simulink model "multirotorPathDynamics"  (R2021b)
settings: Solver=VariableStepAuto  StartTime=0.0  StopTime=210  RelTol=1e-3
InitFcn:
  | FidelityStage = 2;
model workspace (MAT data in the model file):
  airspeedVal = 52.6655095712
  lastWaypointInstance = [-815.416609718; 1327.32979057; -188.3664]
  waypointData = [-1257.59078698 -1257.11235464 -1256.63393535 -1256.15552911 -1255.67713593 -1255.19875581 -1254.72038874 -1254.24203473 -1253.76369377 -1253.28536587 -1252.8070545 -1252.32876157 ... (1797 elements, 599x3)]
undefined symbols (not defined in the file): DroneMass, Dz, Earth, Gravity, Iz, Nz, Pz, startFlightTime, UAVSampleTime, WGS84
libraries: slpidlib x6, uavalgslib x2, aerolibconvert2 x1, aerolibtransform2 x1
(part 1 of 2)
settings Model: DataDictionary=multirotorPathDataDict.sldd  PauseTimes=120  Creator=IRC  LastModifiedBy=IRC
settings DataIOCC: SaveState=on  ReturnWorkspaceOutputs=off
settings DebuggingCC: UnderSpecifiedDataTypeMsg=warning  UnderSpecifiedDimensionMsg=warning

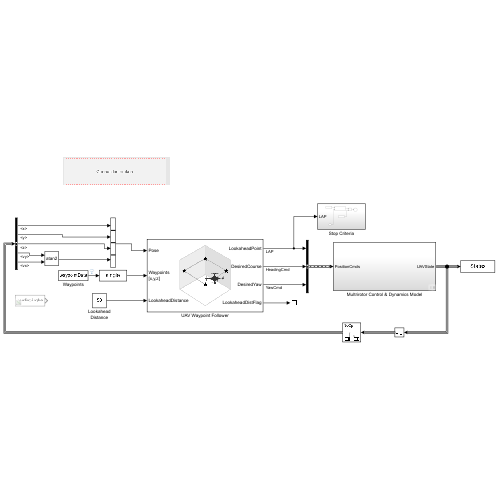
[thumbnail: Simulink's stored preview of the top-level diagram]
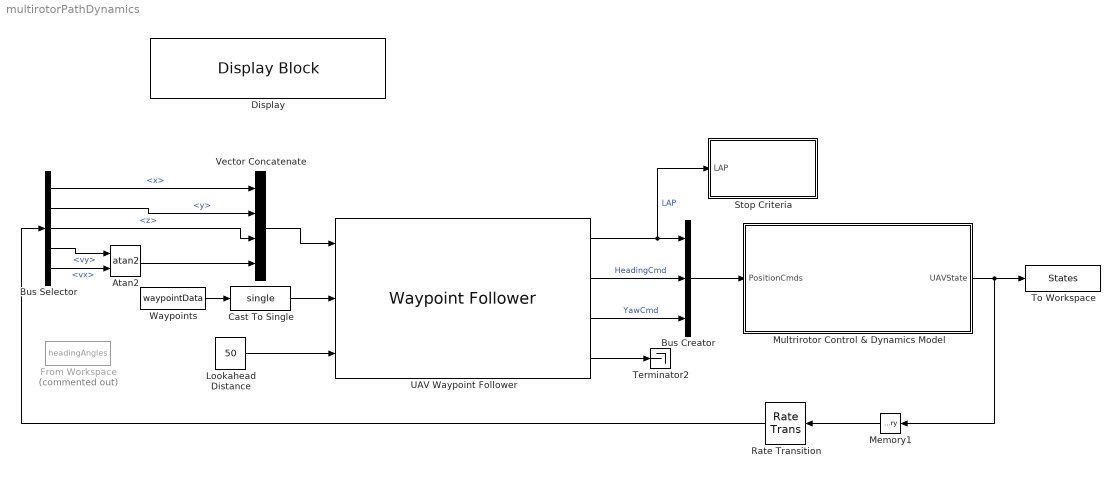
== system multirotorPathDynamics ==
  Atan2 : Trigonometry  Operator=atan2
  Bus Creator : BusCreator  Inputs=3  OutDataTypeStr=Bus: innerLoopCmdsBus  NonVirtualBus=on
  Bus Selector : BusSelector  OutputSignals=pos_vel.x,pos_vel.y,pos_vel.z,pos_vel.vy,pos_vel.vx
  Cast To Single : DataTypeConversion  OutDataTypeStr=single
  Display : DisplayBlock  Format=short  Transparency=1
  From Workspace : FromWorkspace  Commented=on  VariableName=headingAngles  SampleTime=-1
  Lookahead Distance : Constant  Value=50  OutDataTypeStr=single
  Memory1 : Memory  InheritSampleTime=on
  Multrirotor Control & Dynamics Model : Subsystem  VariantControl=plantModelFi ==0
  Rate Transition : RateTransition
  Stop Criteria : Subsystem
  Terminator2 : Terminator
  To Workspace : ToWorkspace  VariableName=States  SaveFormat=Timeseries  SampleTime=-1
  UAV Waypoint Follower : uavalgslib/Waypoint Follower  UAVType=multirotor  StartFrom=first  TransitionRadiusSource=internal  TransitionRadius=10  MinLookaheadDistance=0.1  YawInput=off  ShowCrossTrackErrorOutput=off  ShowStatusOutput=off  SimulateUsing=Code generation
      settings: SourceProductBaseCode=UV
  Vector Concatenate : Concatenate  NumInputs=4
  Waypoints : Constant  Value=waypointData  VectorParams1D=off
  wires:
  UAV Waypoint Follower/1 -> Stop Criteria/1(LAP), Bus Creator/1  "LAP"
  UAV Waypoint Follower/2 -> Bus Creator/2  "HeadingCmd"
  UAV Waypoint Follower/3 -> Bus Creator/3  "YawCmd"
  Lookahead Distance/1 -> UAV Waypoint Follower/3
  Bus Selector/1 -> Vector Concatenate/1  "<x>"
  Bus Selector/2 -> Vector Concatenate/2  "<y>"
  UAV Waypoint Follower/4 -> Terminator2/1
  Waypoints/1 -> Cast To Single/1
  Cast To Single/1 -> UAV Waypoint Follower/2
  Bus Selector/3 -> Vector Concatenate/3  "<z>"
  Vector Concatenate/1 -> UAV Waypoint Follower/1
  Memory1/1 -> Rate Transition/1
  Rate Transition/1 -> Bus Selector/1
  Bus Selector/4 -> Atan2/1  "<vy>"
  Bus Selector/5 -> Atan2/2  "<vx>"
  Atan2/1 -> Vector Concatenate/4
  Bus Creator/1 -> Multrirotor Control & Dynamics Model/1(PositionCmds)
  Multrirotor Control & Dynamics Model/1(UAVState) -> To Workspace/1, Memory1/1

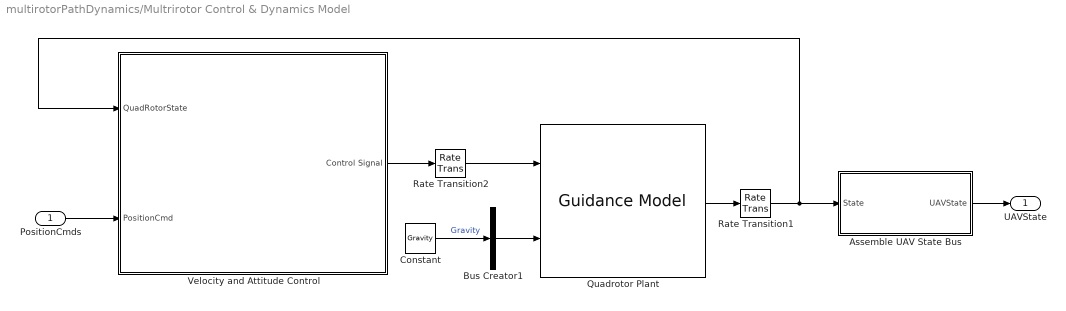
== system multirotorPathDynamics/Multrirotor Control & Dynamics Model ==
  PositionCmds : Inport
  Assemble UAV State Bus : Subsystem
  Bus Creator1 : BusCreator  Inputs=1  OutDataTypeStr=Bus: uavGuidanceEnvironmentBus  NonVirtualBus=on
  Constant : Constant  Value=Gravity  OutDataTypeStr=single
      settings: AttributesFormatString=%<Value>
  Quadrotor Plant : uavalgslib/Guidance Model  ModelType=MultirotorGuidance  SpecifiedDataType=single  SimulateUsing=Code generation  InitialWorldPositionMultirotor=initialConditions.posNED'  InitialWorldVelocityMultirotor=initialConditions.vb'  InitialEulerZYXMultirotor=[0; 0; 0]  InitialBodyAngularRateRPYMultirotor=[0; 0; 0]  InitialThrustMultirotor=0  InitialNorthFixedWing=0  InitialEastFixedWing=0  InitialHeightFixedWing=0  InitialAirSpeedFixedWing=0  InitialHeadingAngleFixedWing=0  InitialFlightPathAngleFixedWing=0  InitialRollAngleFixedWing=0  InitialRollAngleRateFixedWing=0  PDRollMultirotor=[3402.97,116.67]  PDPitchMultirotor=[3402.97, 116.67]  PYawRateMultirotor=1950  PThrustMultirotor=39  MassMultirotor=0.1  PHeightFixedWing=3.9  PHeadingAngleFixedWing=3.9  PFlightPathAngleFixedWing=39  PDRollFixedWing=[3402.97, 116.67]  PAirSpeedFixedWing=1  FlightPathAngleLimitsFixedWing=[-pi/2, pi/2]  StateBusName='uavGuidanceStateBus'  ControlBusName='uavGuidanceControlBus'  EnvironmentBusName='uavGuidanceEnvironmentBus'  DataType=single
      settings: SourceProductName=UAV Toolbox
  Rate Transition1 : RateTransition  OutPortSampleTime=UAVSampleTime
  Rate Transition2 : RateTransition  OutPortSampleTime=UAVSampleTime
  Velocity and Attitude Control : Subsystem
  UAVState : Outport  OutDataTypeStr=Bus: uavStateBus
  wires:
  Constant/1 -> Bus Creator1/1  "Gravity"
  Bus Creator1/1 -> Quadrotor Plant/2
  Velocity and Attitude Control/1(Control Signal) -> Rate Transition2/1
  Quadrotor Plant/1 -> Rate Transition1/1
  Rate Transition2/1 -> Quadrotor Plant/1
  PositionCmds/1 -> Velocity and Attitude Control/2(PositionCmd)
  Rate Transition1/1 -> Velocity and Attitude Control/1(QuadRotorState), Assemble UAV State Bus/1(State)
  Assemble UAV State Bus/1(UAVState) -> UAVState/1

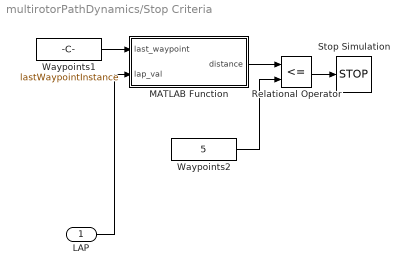
== system multirotorPathDynamics/Stop Criteria ==
  LAP : Inport
  MATLAB Function : MATLAB Function  TreatAsAtomicUnit=on
  Relational Operator : RelationalOperator  Operator=<=  OutDataTypeStr=boolean  RndMeth=Simplest
  Stop Simulation : Stop
  Waypoints1 : Constant  Value=lastWaypointInstance  VectorParams1D=off
  Waypoints2 : Constant  Value=5  VectorParams1D=off
  wires:
  MATLAB Function/1(distance) -> Relational Operator/1
  Waypoints2/1 -> Relational Operator/2
  Waypoints1/1 -> MATLAB Function/1(last_waypoint)
  Relational Operator/1 -> Stop Simulation/1
  LAP/1 -> MATLAB Function/2(lap_val)

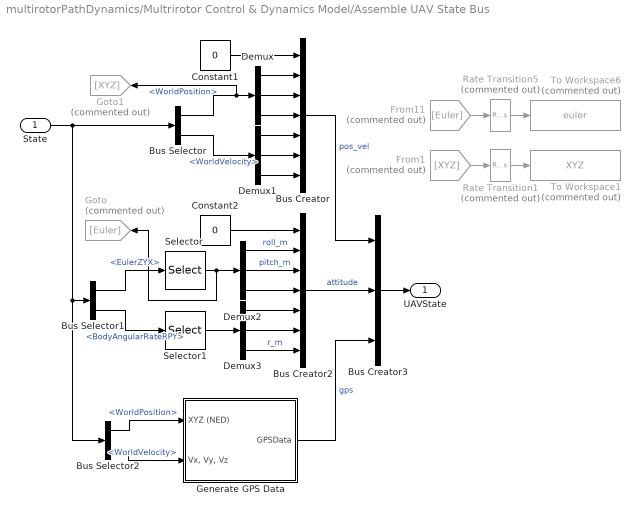
== system multirotorPathDynamics/Multrirotor Control & Dynamics Model/Assemble UAV State Bus ==
  State : Inport
  Bus Creator : BusCreator  Inputs=7  OutDataTypeStr=Bus: local_position_ned
      settings: InheritFromInputs=off
  Bus Creator2 : BusCreator  Inputs=7  OutDataTypeStr=Bus: attitudeBus
      settings: InheritFromInputs=off
  Bus Creator3 : BusCreator  Inputs=3  OutDataTypeStr=Bus: uavStateBus
      settings: InheritFromInputs=off
  Bus Selector : BusSelector  OutputSignals=WorldPosition,WorldVelocity
  Bus Selector1 : BusSelector  OutputSignals=EulerZYX,BodyAngularRateRPY
  Bus Selector2 : BusSelector  OutputSignals=WorldPosition,WorldVelocity
  Constant1 : Constant  Value=0  OutDataTypeStr=uint32
  Constant2 : Constant  Value=0  OutDataTypeStr=uint32
  Demux{,1..3} (4 alike) : Demux  Outputs=3
  From1 : From  Commented=on  GotoTag=XYZ
  From11 : From  Commented=on  GotoTag=Euler
  Generate GPS Data : Subsystem
  Goto : Goto  Commented=on  GotoTag=Euler
  Goto1 : Goto  Commented=on  GotoTag=XYZ
  Rate Transition1 : RateTransition  Commented=on  OutPortSampleTime=UAVSampleTime
  Rate Transition5 : RateTransition  Commented=on  OutPortSampleTime=UAVSampleTime
  Selector : Selector  InputPortWidth=3  IndexOptions=Index vector (dialog)  Indices=[3 2 1]  OutputSizes=1
  Selector1 : Selector  InputPortWidth=3  IndexOptions=Index vector (dialog)  Indices=[3 2 1]  OutputSizes=1
  To Workspace1 : ToWorkspace  Commented=on  VariableName=XYZ  SaveFormat=Timeseries  SampleTime=-1
  To Workspace6 : ToWorkspace  Commented=on  VariableName=euler  SaveFormat=Timeseries  SampleTime=-1
  UAVState : Outport  OutDataTypeStr=Bus: uavStateBus
  wires:
  Bus Creator2/1 -> Bus Creator3/2  "attitude"
  Bus Creator3/1 -> UAVState/1
  Demux3/1 -> Bus Creator2/5
  Demux1/2 -> Bus Creator/6
  Bus Creator/1 -> Bus Creator3/1  "pos_vel"
  Demux1/3 -> Bus Creator/7
  Bus Selector2/2 -> Generate GPS Data/2("Vx, Vy, Vz")  "<WorldVelocity>"
  Demux/1 -> Bus Creator/2
  State/1 -> Bus Selector/1, Bus Selector2/1, Bus Selector1/1
  Constant2/1 -> Bus Creator2/1
  Bus Selector/1 -> Goto1/1, Demux/1  "<WorldPosition>"
  Selector1/1 -> Demux3/1
  Demux1/1 -> Bus Creator/5
  Bus Selector1/1 -> Selector/1  "<EulerZYX>"
  Demux/2 -> Bus Creator/3
  Demux2/1 -> Bus Creator2/2  "roll_m"
  Demux2/3 -> Bus Creator2/4
  Demux3/2 -> Bus Creator2/6
  Demux2/2 -> Bus Creator2/3  "pitch_m"
  Bus Selector1/2 -> Selector1/1  "<BodyAngularRateRPY>"
  Demux3/3 -> Bus Creator2/7  "r_m"
  Demux/3 -> Bus Creator/4
  Bus Selector/2 -> Demux1/1  "<WorldVelocity>"
  Constant1/1 -> Bus Creator/1
  Bus Selector2/1 -> Generate GPS Data/1(XYZ (NED))  "<WorldPosition>"
  Generate GPS Data/1(GPSData) -> Bus Creator3/3  "gps"
  Rate Transition5/1 -> To Workspace6/1
  From11/1 -> Rate Transition5/1
  Selector/1 -> Goto/1, Demux2/1
  From1/1 -> Rate Transition1/1
  Rate Transition1/1 -> To Workspace1/1

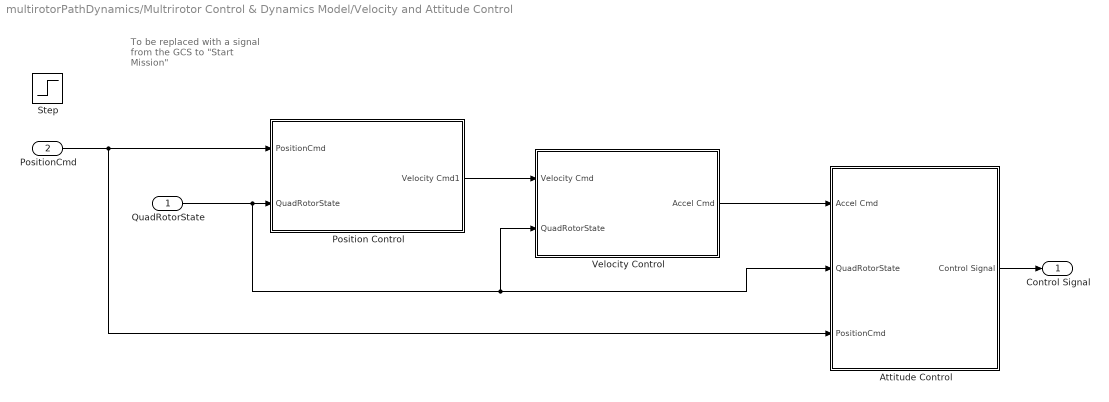
== system multirotorPathDynamics/Multrirotor Control & Dynamics Model/Velocity and Attitude Control ==
  note: To be replaced with a signal from the GCS to "Start Mission"
  QuadRotorState : Inport
  PositionCmd : Inport  Port=2
  Attitude Control : Subsystem
  Position Control : Subsystem
  Step : Step  Time=startFlightTime  SampleTime=UAVSampleTime
  Velocity Control : Subsystem
  Control Signal : Outport
  wires:
  PositionCmd/1 -> Position Control/1(PositionCmd), Attitude Control/3(PositionCmd)
  Velocity Control/1(Accel Cmd) -> Attitude Control/1(Accel Cmd)
  Attitude Control/1(Control Signal) -> Control Signal/1
  QuadRotorState/1 -> Velocity Control/2(QuadRotorState), Attitude Control/2(QuadRotorState), Position Control/2(QuadRotorState)
  Position Control/1(Velocity Cmd1) -> Velocity Control/1(Velocity Cmd)

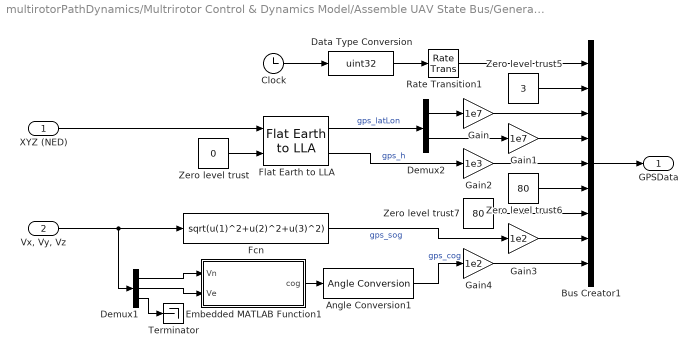
== system multirotorPathDynamics/Multrirotor Control & Dynamics Model/Assemble UAV State Bus/Generate GPS Data ==
  XYZ (NED) : Inport
  "Vx, Vy, Vz" : Inport  Port=2
  Angle Conversion1 : aerolibconvert2/Angle Conversion  IU=rad  OU=deg
  Bus Creator1 : BusCreator  Inputs=9  OutDataTypeStr=Bus: gps_raw_int  NonVirtualBus=on
      settings: InheritFromInputs=off
  Clock : Clock
      settings: AttributesFormatString=Decimation: %<Decimation>
  Data Type Conversion : DataTypeConversion  OutDataTypeStr=uint32
  Demux1 : Demux  Outputs=3
  Demux2 : Demux  Outputs=2
  Embedded MATLAB Function1 : MATLAB Function  TreatAsAtomicUnit=on
  Fcn : Fcn  Expr=sqrt(u(1)^2+u(2)^2+u(3)^2)
  Flat Earth to LLA : aerolibtransform2/Flat Earth to LLA  units=Metric (MKS)  ptype=Earth (WGS84)  F=1/298.257223563  R=6378137  refPosPort=off  LL0=uavIC_latLon  psi=0
  Gain : Gain  Gain=1e7  OutDataTypeStr=int32
  Gain1 : Gain  Gain=1e7  OutDataTypeStr=int32
  Gain2 : Gain  Gain=1e3  OutDataTypeStr=int32
  Gain3 : Gain  Gain=1e2  OutDataTypeStr=uint16
  Gain4 : Gain  Gain=1e2  OutDataTypeStr=uint16
  Rate Transition1 : RateTransition  OutPortSampleTime=UAVSampleTime
  Terminator : Terminator
  Zero level trust : Constant  Value=0
      settings: AttributesFormatString=%<Value>
  Zero level trust5 : Constant  Value=3  OutDataTypeStr=uint8
      settings: AttributesFormatString=%<Value>
  Zero level trust6 : Constant  Value=80  OutDataTypeStr=uint16
      settings: AttributesFormatString=%<Value>
  Zero level trust7 : Constant  Value=80  OutDataTypeStr=uint16
      settings: AttributesFormatString=%<Value>
  GPSData : Outport  VectorParamsAs1DForOutWhenUnconnected=off
  wires:
  Demux1/3 -> Terminator/1
  Angle Conversion1/1 -> Gain4/1  "gps_cog"
  Embedded MATLAB Function1/1(cog) -> Angle Conversion1/1
  "Vx, Vy, Vz"/1 -> Demux1/1, Fcn/1
  Demux1/2 -> Embedded MATLAB Function1/2(Ve)
  Demux1/1 -> Embedded MATLAB Function1/1(Vn)
  Fcn/1 -> Gain3/1  "gps_sog"
  Flat Earth to LLA/1 -> Demux2/1  "gps_latLon"
  Zero level trust/1 -> Flat Earth to LLA/2
  XYZ (NED)/1 -> Flat Earth to LLA/1
  Clock/1 -> Data Type Conversion/1
  Flat Earth to LLA/2 -> Gain2/1  "gps_h"
  Demux2/1 -> Gain/1
  Demux2/2 -> Gain1/1
  Zero level trust5/1 -> Bus Creator1/2
  Gain1/1 -> Bus Creator1/4
  Zero level trust6/1 -> Bus Creator1/6
  Gain3/1 -> Bus Creator1/8
  Zero level trust7/1 -> Bus Creator1/7
  Gain4/1 -> Bus Creator1/9
  Gain2/1 -> Bus Creator1/5
  Gain/1 -> Bus Creator1/3
  Data Type Conversion/1 -> Rate Transition1/1
  Bus Creator1/1 -> GPSData/1
  Rate Transition1/1 -> Bus Creator1/1

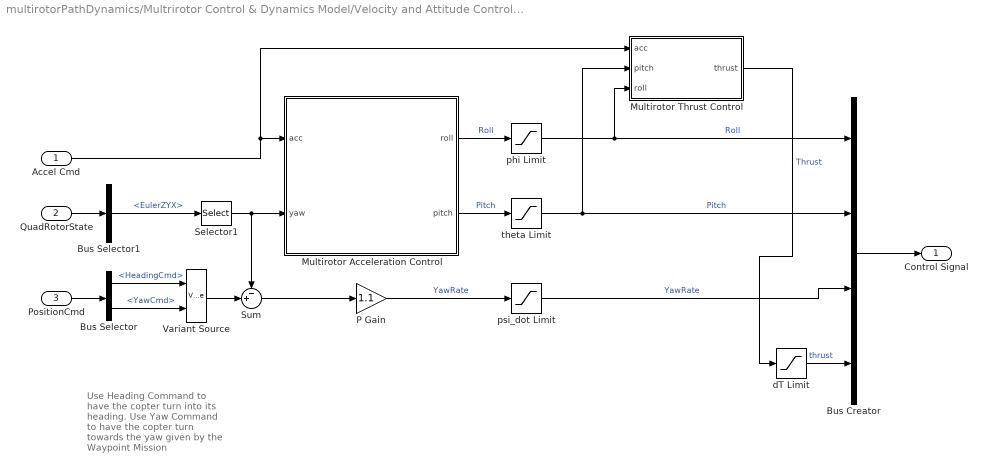
== system multirotorPathDynamics/Multrirotor Control & Dynamics Model/Velocity and Attitude Control/Attitude Control ==
  note: Use Heading Command to have
      | the copter turn into its heading.
      | Use Yaw Command to have the
      | copter turn towards the yaw given
      | by the Waypoint Mission
  Accel Cmd : Inport
  QuadRotorState : Inport  Port=2
  PositionCmd : Inport  Port=3
  Bus Creator : BusCreator  Inputs=4  OutDataTypeStr=Bus: uavGuidanceControlBus  NonVirtualBus=on
      settings: InheritFromInputs=off
  Bus Selector : BusSelector  OutputSignals=HeadingCmd,YawCmd
  Bus Selector1 : BusSelector  OutputSignals=EulerZYX
  Multirotor Acceleration Control : MATLAB Function  TreatAsAtomicUnit=on
  Multirotor Thrust Control : MATLAB Function  TreatAsAtomicUnit=on
  P Gain : Gain  Gain=1.1
  Selector1 : Selector  InputPortWidth=3  IndexOptions=Index vector (dialog)  Indices=[1]  OutputSizes=1
  Sum : Sum  Inputs=-+|
  Variant Source : VariantSource
  dT Limit : Saturate  UpperLimit=1.2  LowerLimit=0
      settings: AttributesFormatString=[%<UpperLimit> %<LowerLimit>]
  phi Limit : Saturate  UpperLimit=25*pi/180  LowerLimit=-25*pi/180
      settings: AttributesFormatString=[%<UpperLimit> %<LowerLimit>]
  psi_dot Limit : Saturate  UpperLimit=30*pi/180  LowerLimit=-30*pi/180
      settings: AttributesFormatString=[%<UpperLimit> %<LowerLimit>]
  theta Limit : Saturate  UpperLimit=25*pi/180  LowerLimit=-25*pi/180
      settings: AttributesFormatString=[%<UpperLimit> %<LowerLimit>]
  Control Signal : Outport
  wires:
  Multirotor Thrust Control/1(thrust) -> dT Limit/1  "Thrust"
  QuadRotorState/1 -> Bus Selector1/1
  Multirotor Acceleration Control/1(roll) -> phi Limit/1  "Roll"
  Bus Creator/1 -> Control Signal/1
  dT Limit/1 -> Bus Creator/4  "thrust"
  P Gain/1 -> psi_dot Limit/1  "YawRate"
  Accel Cmd/1 -> Multirotor Thrust Control/1(acc), Multirotor Acceleration Control/1(acc)
  theta Limit/1 -> Bus Creator/2, Multirotor Thrust Control/2(pitch)  "Pitch"
  Sum/1 -> P Gain/1
  Selector1/1 -> Sum/1, Multirotor Acceleration Control/2(yaw)
  psi_dot Limit/1 -> Bus Creator/3  "YawRate"
  Bus Selector/2 -> Variant Source/2  "<YawCmd>"
  phi Limit/1 -> Bus Creator/1, Multirotor Thrust Control/3(roll)  "Roll"
  Variant Source/1 -> Sum/2
  Bus Selector1/1 -> Selector1/1  "<EulerZYX>"
  PositionCmd/1 -> Bus Selector/1
  Multirotor Acceleration Control/2(pitch) -> theta Limit/1  "Pitch"
  Bus Selector/1 -> Variant Source/1  "<HeadingCmd>"
